simulink model "dexter_dsp_tx"  (R2020a)
settings: Solver=VariableStepAuto  StartTime=0.0  StopTime=5e4/clk  RelTol=1e-3
InitFcn:
  | dexter_dsp_init
values from neighbouring files (symbols this model uses):
  a_stimulus = [0.5 0.00 0.000]    [dexter_dsp_init.m]
  clk = 163.84e6    (= 163840000)    [dexter_dsp_init.m]
  f_stimulus = [100000 700000 768000]    [dexter_dsp_init.m]
  fs_dab = 2048e3    (= 2048000)    [dexter_dsp_init.m]
  fs_dac = clk/2    (= 81920000)    [dexter_dsp_init.m]
  interp = fir_interpolation*hb_interpolation    (= 40)    [dexter_dsp_init.m]
  tx_inc = mod(round(tx_dds_freq*2^dds_phasewidth/clk*2),2^dds_phasewidth)    [dexter_dsp_init.m]
undefined symbols (not defined in the file or in its folder): AXI4, Lite
libraries: xbsIndex_r4 x210, dspsrcs4 x1
(part 1 of 3)
settings Model: Creator=zta1  LastModifiedBy=zta1

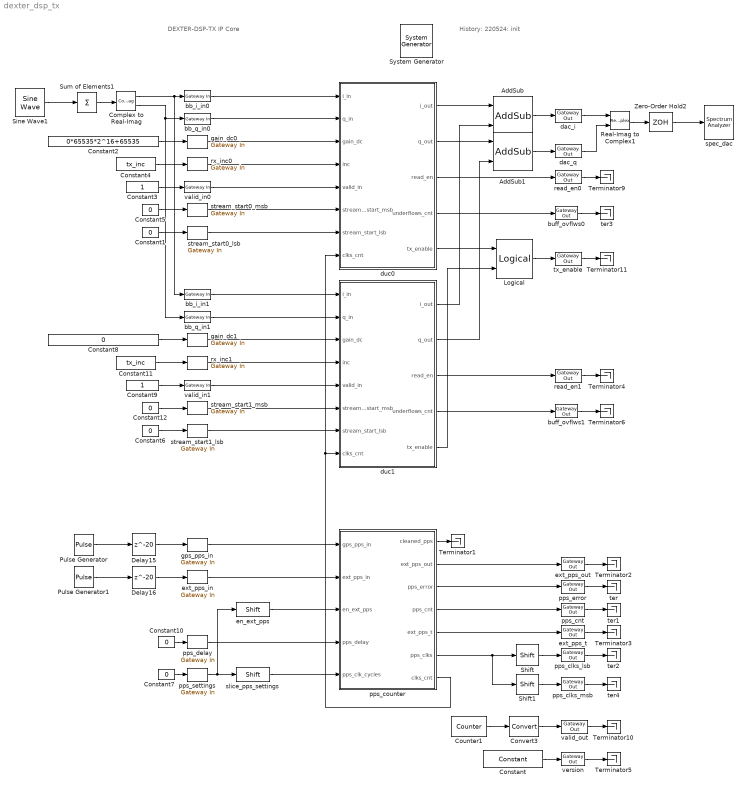
== system dexter_dsp_tx ==
  note: History:
      | 220524: init
  note: DEXTER-DSP-TX IP Core
  " System Generator" : xbsIndex_r4/ System Generator  Tag=genX  xilinxfamily=zynq  part=xc7z020  speed=-2  package=clg400  synthesis_tool=Vivado  clock_wrapper=Clock Enables  directory=../library/dexter_dsp_tx  proj_type=Vivado  Synth_file=Vivado Synthesis Defaults  Impl_file=Vivado Implementation Defaults  testbench=off  simulink_period=1/clk  sysclk_period=1e9/clk  dcm_input_clock_period=10  incr_netlist=off  trim_vbits=Everywhere in SubSystem  dbl_ovrd=According to Block Masks  core_generation=According to Block Masks  run_coregen=off  deprecated_control=off  eval_field=0  block_type=sysgen
  AddSub : xbsIndex_r4/AddSub  mode=Addition  use_carryin=off  use_carryout=off  en=off  latency=3  precision=User Defined  arith_type="Signed  (2's comp)"  n_bits=18  bin_pt=17  quantization="Round  (unbiased: +/- Inf)"  overflow=Saturate  use_behavioral_HDL=off  hw_selection=Fabric  pipelined=off  dbl_ovrd=off  block_type=addsub
  AddSub1 : xbsIndex_r4/AddSub  mode=Addition  use_carryin=off  use_carryout=off  en=off  latency=3  precision=User Defined  arith_type="Signed  (2's comp)"  n_bits=18  bin_pt=17  quantization="Round  (unbiased: +/- Inf)"  overflow=Saturate  use_behavioral_HDL=off  hw_selection=Fabric  pipelined=off  dbl_ovrd=off  block_type=addsub
  Complex to Real-Imag : ComplexToRealImag
  Constant : xbsIndex_r4/Constant  const=220524  gui_display_data_type=Fixed-point  arith_type=Unsigned  n_bits=32  bin_pt=0  preci_type=Single  exp_width=8  frac_width=24  explicit_period=on  period=1/clk  equ=P=C  opselect=C  inp2=PCIN>>17  opr=+  inp1=P  carry=CIN  dbl_ovrd=off  block_type=constant
  Constant{1,5..7,10,12} (6 alike) : Constant  Value=0  OutDataTypeStr=fixdt(0,32,0)
  Constant11 : Constant  Value=tx_inc
  Constant2 : Constant  Value=0*65535*2^16+65535  OutDataTypeStr=uint32
  Constant3 : Constant
  Constant4 : Constant  Value=tx_inc
  Constant8 : Constant  Value=0  OutDataTypeStr=uint32
  Constant9 : Constant
  Convert3 : xbsIndex_r4/Convert  gui_display_data_type=Boolean  arith_type=Boolean  n_bits=1  bin_pt=0  float_type=Single  exp_bits=8  fraction_bits=24  quantization=Truncate  overflow=Wrap  en=off  latency=0  pipeline=off  dbl_ovrd=off  block_type=convert
  Counter1 : xbsIndex_r4/Counter  cnt_type=Free Running  cnt_to=Inf  operation=Up  start_count=0  cnt_by_val=1  arith_type=Unsigned  n_bits=1  bin_pt=0  load_pin=off  rst=off  en=off  explicit_period=on  period=1/clk  use_behavioral_HDL=off  implementation=Fabric  dbl_ovrd=off  block_type=counter
  Delay15 : Delay  DelayLength=20
  Delay16 : Delay  DelayLength=20
  Logical : xbsIndex_r4/Logical  logical_function=OR  inputs=2  en=off  latency=1  precision=Full  arith_type=Unsigned  n_bits=16  bin_pt=0  align_bp=on  dbl_ovrd=off  block_type=logical
  Pulse Generator : DiscretePulseGenerator  Period=500  PulseWidth=5  SampleTime=1/clk
  Pulse Generator1 : DiscretePulseGenerator  Period=200  PulseWidth=5  SampleTime=1/clk
  Real-Imag to Complex1 : RealImagToComplex
  Shift : xbsIndex_r4/Shift  shift_dir=Right  shift_bits=0  en=off  latency=1  precision=User Defined  arith_type=Unsigned  n_bits=32  bin_pt=0  quantization=Truncate  overflow=Wrap  dbl_ovrd=off  block_type=shift
  Shift1 : xbsIndex_r4/Shift  shift_dir=Right  shift_bits=32  en=off  latency=1  precision=User Defined  arith_type=Unsigned  n_bits=32  bin_pt=0  quantization=Truncate  overflow=Wrap  dbl_ovrd=off  block_type=shift
  Sine Wave1 : dspsrcs4/Sine Wave  Amplitude=a_stimulus  Frequency=f_stimulus  Phase=0  SampleMode=Discrete  OutComplex=Complex  CompMethod=Trigonometric fcn  TableSize=Speed  SampleTime=1/fs_dab  SamplesPerFrame=1  ResetState=Restart at time zero  OutputFrames=off  dataType=double  wordLen=16  udDataType=sfix(16)  fracBitsMode=Best precision  numFracBits=15  OutDataTypeStr=double  LastOutDataTypeStr=double
  Sum of Elements1 : Sum  Inputs=+
  Terminator{1..6,9..11} (9 alike) : Terminator
  Zero-Order Hold2 : ZeroOrderHold  SampleTime=1/fs_dac
  bb_i_in0 : xbsIndex_r4/Gateway In  gui_display_data_type=Fixed-point  arith_type="Signed  (2's comp)"  n_bits=16  bin_pt=15  preci_type=Single  exp_width=8  frac_width=24  rows=1  columns=1  quantization="Round  (unbiased: +/- Inf)"  overflow=Wrap  period=1/fs_dab  UseAsADC=off  ADCChannel='1'  interface=None  automatic_assignment=on  address_offset=hex2dec('00')  intf_name=''  intf_description=''  default_value=0  timing_constraint=None  locs_specified=off  LOCs={}  io_standard={}  inherit_from_input=off  hdl_port=on  dbl_ovrd=off  block_type=gatewayin
  bb_i_in1 : xbsIndex_r4/Gateway In  gui_display_data_type=Fixed-point  arith_type="Signed  (2's comp)"  n_bits=16  bin_pt=15  preci_type=Single  exp_width=8  frac_width=24  rows=1  columns=1  quantization="Round  (unbiased: +/- Inf)"  overflow=Wrap  period=1/fs_dab  UseAsADC=off  ADCChannel='1'  interface=None  automatic_assignment=on  address_offset=hex2dec('00')  intf_name=''  intf_description=''  default_value=0  timing_constraint=None  locs_specified=off  LOCs={}  io_standard={}  inherit_from_input=off  hdl_port=on  dbl_ovrd=off  block_type=gatewayin
  bb_q_in0 : xbsIndex_r4/Gateway In  gui_display_data_type=Fixed-point  arith_type="Signed  (2's comp)"  n_bits=16  bin_pt=15  preci_type=Single  exp_width=8  frac_width=24  rows=1  columns=1  quantization="Round  (unbiased: +/- Inf)"  overflow=Wrap  period=1/fs_dab  UseAsADC=off  ADCChannel='1'  interface=None  automatic_assignment=on  address_offset=hex2dec('00')  intf_name=''  intf_description=''  default_value=0  timing_constraint=None  locs_specified=off  LOCs={}  io_standard={}  inherit_from_input=off  hdl_port=on  dbl_ovrd=off  block_type=gatewayin
  bb_q_in1 : xbsIndex_r4/Gateway In  gui_display_data_type=Fixed-point  arith_type="Signed  (2's comp)"  n_bits=16  bin_pt=15  preci_type=Single  exp_width=8  frac_width=24  rows=1  columns=1  quantization="Round  (unbiased: +/- Inf)"  overflow=Wrap  period=1/fs_dab  UseAsADC=off  ADCChannel='1'  interface=None  automatic_assignment=on  address_offset=hex2dec('00')  intf_name=''  intf_description=''  default_value=0  timing_constraint=None  locs_specified=off  LOCs={}  io_standard={}  inherit_from_input=off  hdl_port=on  dbl_ovrd=off  block_type=gatewayin
  buff_ovflws0 : xbsIndex_r4/Gateway Out  inherit_from_input=off  hdl_port=on  rows=1  columns=1  UseAsDAC=off  DACChannel='1'  interface=AXI4-Lite  automatic_assignment=off  address_offset=4*18  intf_name=''  intf_description=''  timing_constraint=None  locs_specified=off  LOCs={}  io_standard={}  block_type=gatewayout
  buff_ovflws1 : xbsIndex_r4/Gateway Out  inherit_from_input=off  hdl_port=on  rows=1  columns=1  UseAsDAC=off  DACChannel='1'  interface=AXI4-Lite  automatic_assignment=off  address_offset=4*34  intf_name=''  intf_description=''  timing_constraint=None  locs_specified=off  LOCs={}  io_standard={}  block_type=gatewayout
  dac_i : xbsIndex_r4/Gateway Out  inherit_from_input=off  hdl_port=on  rows=1  columns=1  UseAsDAC=off  DACChannel='1'  interface=None  automatic_assignment=on  address_offset=hex2dec('00')  intf_name=''  intf_description=''  timing_constraint=None  locs_specified=off  LOCs={}  io_standard={}  block_type=gatewayout
  dac_q : xbsIndex_r4/Gateway Out  inherit_from_input=off  hdl_port=on  rows=1  columns=1  UseAsDAC=off  DACChannel='1'  interface=None  automatic_assignment=on  address_offset=hex2dec('00')  intf_name=''  intf_description=''  timing_constraint=None  locs_specified=off  LOCs={}  io_standard={}  block_type=gatewayout
  duc0 : Subsystem
  duc1 : Subsystem
  en_ext_pps : xbsIndex_r4/Shift  shift_dir=Right  shift_bits=29  en=off  latency=0  precision=User Defined  arith_type=Unsigned  n_bits=1  bin_pt=0  quantization=Truncate  overflow=Wrap  dbl_ovrd=off  block_type=shift
      settings: xl_area=[0 0 0 0 0 0 0]
  ext_pps_in : xbsIndex_r4/Gateway In  gui_display_data_type=Boolean  arith_type=Boolean  n_bits=16  bin_pt=15  preci_type=Single  exp_width=8  frac_width=24  rows=1  columns=1  quantization="Round  (unbiased: +/- Inf)"  overflow=Wrap  period=1/clk  UseAsADC=off  ADCChannel='1'  interface=None  automatic_assignment=on  address_offset=hex2dec('00')  intf_name=''  intf_description=''  default_value=0  timing_constraint=None  locs_specified=off  LOCs={}  io_standard={}  inherit_from_input=off  hdl_port=on  dbl_ovrd=off  block_type=gatewayin
  ext_pps_out : xbsIndex_r4/Gateway Out  inherit_from_input=off  hdl_port=on  rows=1  columns=1  UseAsDAC=off  DACChannel='1'  interface=None  automatic_assignment=off  address_offset=10*4  intf_name=''  intf_description=''  timing_constraint=None  locs_specified=off  LOCs={}  io_standard={}  block_type=gatewayout
  ext_pps_t : xbsIndex_r4/Gateway Out  inherit_from_input=off  hdl_port=on  rows=1  columns=1  UseAsDAC=off  DACChannel='1'  interface=None  automatic_assignment=off  address_offset=10*4  intf_name=''  intf_description=''  timing_constraint=None  locs_specified=off  LOCs={}  io_standard={}  block_type=gatewayout
  gain_dc0 : xbsIndex_r4/Gateway In  gui_display_data_type=Fixed-point  arith_type=Unsigned  n_bits=32  bin_pt=0  preci_type=Single  exp_width=8  frac_width=24  rows=1  columns=1  quantization=Truncate  overflow=Wrap  period=1/fs_dab  UseAsADC=off  ADCChannel='1'  interface=AXI4-Lite  automatic_assignment=off  address_offset=4*17  intf_name=''  intf_description=''  default_value=0  timing_constraint=None  locs_specified=off  LOCs={}  io_standard={}  inherit_from_input=off  hdl_port=on  dbl_ovrd=off  block_type=gatewayin
      settings: xl_area=[0 0 0 0 32 0 0]
  gain_dc1 : xbsIndex_r4/Gateway In  gui_display_data_type=Fixed-point  arith_type=Unsigned  n_bits=32  bin_pt=0  preci_type=Single  exp_width=8  frac_width=24  rows=1  columns=1  quantization=Truncate  overflow=Wrap  period=1/fs_dab  UseAsADC=off  ADCChannel='1'  interface=AXI4-Lite  automatic_assignment=off  address_offset=4*33  intf_name=''  intf_description=''  default_value=0  timing_constraint=None  locs_specified=off  LOCs={}  io_standard={}  inherit_from_input=off  hdl_port=on  dbl_ovrd=off  block_type=gatewayin
      settings: xl_area=[0 0 0 0 32 0 0]
  gps_pps_in : xbsIndex_r4/Gateway In  gui_display_data_type=Boolean  arith_type=Boolean  n_bits=16  bin_pt=15  preci_type=Single  exp_width=8  frac_width=24  rows=1  columns=1  quantization="Round  (unbiased: +/- Inf)"  overflow=Wrap  period=1/clk  UseAsADC=off  ADCChannel='1'  interface=None  automatic_assignment=on  address_offset=hex2dec('00')  intf_name=''  intf_description=''  default_value=0  timing_constraint=None  locs_specified=off  LOCs={}  io_standard={}  inherit_from_input=off  hdl_port=on  dbl_ovrd=off  block_type=gatewayin
  pps_clks_lsb : xbsIndex_r4/Gateway Out  inherit_from_input=off  hdl_port=on  rows=1  columns=1  UseAsDAC=off  DACChannel='1'  interface=AXI4-Lite  automatic_assignment=off  address_offset=4*5  intf_name=''  intf_description=''  timing_constraint=None  locs_specified=off  LOCs={}  io_standard={}  block_type=gatewayout
  pps_clks_msb : xbsIndex_r4/Gateway Out  inherit_from_input=off  hdl_port=on  rows=1  columns=1  UseAsDAC=off  DACChannel='1'  interface=AXI4-Lite  automatic_assignment=off  address_offset=4*6  intf_name=''  intf_description=''  timing_constraint=None  locs_specified=off  LOCs={}  io_standard={}  block_type=gatewayout
  pps_cnt : xbsIndex_r4/Gateway Out  inherit_from_input=off  hdl_port=on  rows=1  columns=1  UseAsDAC=off  DACChannel='1'  interface=AXI4-Lite  automatic_assignment=off  address_offset=4*3  intf_name=''  intf_description=''  timing_constraint=None  locs_specified=off  LOCs={}  io_standard={}  block_type=gatewayout
  pps_counter : Subsystem
  pps_delay : xbsIndex_r4/Gateway In  gui_display_data_type=Fixed-point  arith_type=Unsigned  n_bits=29  bin_pt=0  preci_type=Single  exp_width=8  frac_width=24  rows=1  columns=1  quantization=Truncate  overflow=Wrap  period=1/clk  UseAsADC=off  ADCChannel='1'  interface=AXI4-Lite  automatic_assignment=off  address_offset=4*4  intf_name=''  intf_description=''  default_value=0  timing_constraint=None  locs_specified=off  LOCs={}  io_standard={}  inherit_from_input=off  hdl_port=on  dbl_ovrd=off  block_type=gatewayin
      settings: xl_area=[0 0 0 0 32 0 0]
  pps_error : xbsIndex_r4/Gateway Out  inherit_from_input=off  hdl_port=on  rows=1  columns=1  UseAsDAC=off  DACChannel='1'  interface=AXI4-Lite  automatic_assignment=off  address_offset=4*2  intf_name=''  intf_description=''  timing_constraint=None  locs_specified=off  LOCs={}  io_standard={}  block_type=gatewayout
  pps_settings : xbsIndex_r4/Gateway In  gui_display_data_type=Fixed-point  arith_type=Unsigned  n_bits=32  bin_pt=0  preci_type=Single  exp_width=8  frac_width=24  rows=1  columns=1  quantization=Truncate  overflow=Wrap  period=1/clk  UseAsADC=off  ADCChannel='1'  interface=AXI4-Lite  automatic_assignment=off  address_offset=4*1  intf_name=''  intf_description=''  default_value=0  timing_constraint=None  locs_specified=off  LOCs={}  io_standard={}  inherit_from_input=off  hdl_port=on  dbl_ovrd=off  block_type=gatewayin
      settings: xl_area=[0 0 0 0 32 0 0]
  read_en0 : xbsIndex_r4/Gateway Out  inherit_from_input=off  hdl_port=on  rows=1  columns=1  UseAsDAC=off  DACChannel='1'  interface=None  automatic_assignment=on  address_offset=hex2dec('00')  intf_name=''  intf_description=''  timing_constraint=None  locs_specified=off  LOCs={}  io_standard={}  block_type=gatewayout
  read_en1 : xbsIndex_r4/Gateway Out  inherit_from_input=off  hdl_port=on  rows=1  columns=1  UseAsDAC=off  DACChannel='1'  interface=None  automatic_assignment=on  address_offset=hex2dec('00')  intf_name=''  intf_description=''  timing_constraint=None  locs_specified=off  LOCs={}  io_standard={}  block_type=gatewayout
  rx_inc0 : xbsIndex_r4/Gateway In  gui_display_data_type=Fixed-point  arith_type=Unsigned  n_bits=dds_phasewidth  bin_pt=0  preci_type=Single  exp_width=8  frac_width=24  rows=1  columns=1  quantization=Truncate  overflow=Wrap  period=2/clk  UseAsADC=off  ADCChannel='1'  interface=AXI4-Lite  automatic_assignment=off  address_offset=4*16  intf_name=''  intf_description=''  default_value=0  timing_constraint=None  locs_specified=off  LOCs={}  io_standard={}  inherit_from_input=off  hdl_port=on  dbl_ovrd=off  block_type=gatewayin
      settings: xl_area=[0 0 0 0 32 0 0]
  rx_inc1 : xbsIndex_r4/Gateway In  gui_display_data_type=Fixed-point  arith_type=Unsigned  n_bits=dds_phasewidth  bin_pt=0  preci_type=Single  exp_width=8  frac_width=24  rows=1  columns=1  quantization=Truncate  overflow=Wrap  period=2/clk  UseAsADC=off  ADCChannel='1'  interface=AXI4-Lite  automatic_assignment=off  address_offset=4*32  intf_name=''  intf_description=''  default_value=0  timing_constraint=None  locs_specified=off  LOCs={}  io_standard={}  inherit_from_input=off  hdl_port=on  dbl_ovrd=off  block_type=gatewayin
      settings: xl_area=[0 0 0 0 32 0 0]
  slice_pps_settings : xbsIndex_r4/Shift  shift_dir=Right  shift_bits=0  en=off  latency=0  precision=User Defined  arith_type=Unsigned  n_bits=29  bin_pt=0  quantization=Truncate  overflow=Wrap  dbl_ovrd=off  block_type=shift
      settings: xl_area=[0 0 0 0 0 0 0]
  spec_dac : SpectrumAnalyzer
  stream_start0_lsb : xbsIndex_r4/Gateway In  gui_display_data_type=Fixed-point  arith_type=Unsigned  n_bits=32  bin_pt=0  preci_type=Single  exp_width=8  frac_width=24  rows=1  columns=1  quantization=Truncate  overflow=Wrap  period=1/clk  UseAsADC=off  ADCChannel='1'  interface=AXI4-Lite  automatic_assignment=off  address_offset=4*19  intf_name=''  intf_description=''  default_value=0  timing_constraint=None  locs_specified=off  LOCs={}  io_standard={}  inherit_from_input=off  hdl_port=on  dbl_ovrd=off  block_type=gatewayin
      settings: xl_area=[0 0 0 0 32 0 0]
  stream_start0_msb : xbsIndex_r4/Gateway In  gui_display_data_type=Fixed-point  arith_type=Unsigned  n_bits=32  bin_pt=0  preci_type=Single  exp_width=8  frac_width=24  rows=1  columns=1  quantization=Truncate  overflow=Wrap  period=1/clk  UseAsADC=off  ADCChannel='1'  interface=AXI4-Lite  automatic_assignment=off  address_offset=4*20  intf_name=''  intf_description=''  default_value=0  timing_constraint=None  locs_specified=off  LOCs={}  io_standard={}  inherit_from_input=off  hdl_port=on  dbl_ovrd=off  block_type=gatewayin
      settings: xl_area=[0 0 0 0 32 0 0]
  stream_start1_lsb : xbsIndex_r4/Gateway In  gui_display_data_type=Fixed-point  arith_type=Unsigned  n_bits=32  bin_pt=0  preci_type=Single  exp_width=8  frac_width=24  rows=1  columns=1  quantization=Truncate  overflow=Wrap  period=1/clk  UseAsADC=off  ADCChannel='1'  interface=AXI4-Lite  automatic_assignment=off  address_offset=4*35  intf_name=''  intf_description=''  default_value=0  timing_constraint=None  locs_specified=off  LOCs={}  io_standard={}  inherit_from_input=off  hdl_port=on  dbl_ovrd=off  block_type=gatewayin
      settings: xl_area=[0 0 0 0 32 0 0]
  stream_start1_msb : xbsIndex_r4/Gateway In  gui_display_data_type=Fixed-point  arith_type=Unsigned  n_bits=32  bin_pt=0  preci_type=Single  exp_width=8  frac_width=24  rows=1  columns=1  quantization=Truncate  overflow=Wrap  period=1/clk  UseAsADC=off  ADCChannel='1'  interface=AXI4-Lite  automatic_assignment=off  address_offset=4*36  intf_name=''  intf_description=''  default_value=0  timing_constraint=None  locs_specified=off  LOCs={}  io_standard={}  inherit_from_input=off  hdl_port=on  dbl_ovrd=off  block_type=gatewayin
      settings: xl_area=[0 0 0 0 32 0 0]
  ter{,1..4} (5 alike) : Terminator
  tx_enable : xbsIndex_r4/Gateway Out  inherit_from_input=off  hdl_port=on  rows=1  columns=1  UseAsDAC=off  DACChannel='1'  interface=None  automatic_assignment=on  address_offset=hex2dec('00')  intf_name=''  intf_description=''  timing_constraint=None  locs_specified=off  LOCs={}  io_standard={}  block_type=gatewayout
  valid_in0 : xbsIndex_r4/Gateway In  gui_display_data_type=Boolean  arith_type=Boolean  n_bits=16  bin_pt=15  preci_type=Single  exp_width=8  frac_width=24  rows=1  columns=1  quantization="Round  (unbiased: +/- Inf)"  overflow=Wrap  period=1/clk  UseAsADC=off  ADCChannel='1'  interface=None  automatic_assignment=on  address_offset=hex2dec('00')  intf_name=''  intf_description=''  default_value=0  timing_constraint=None  locs_specified=off  LOCs={}  io_standard={}  inherit_from_input=off  hdl_port=on  dbl_ovrd=off  block_type=gatewayin
  valid_in1 : xbsIndex_r4/Gateway In  gui_display_data_type=Boolean  arith_type=Boolean  n_bits=16  bin_pt=15  preci_type=Single  exp_width=8  frac_width=24  rows=1  columns=1  quantization="Round  (unbiased: +/- Inf)"  overflow=Wrap  period=1/clk  UseAsADC=off  ADCChannel='1'  interface=None  automatic_assignment=on  address_offset=hex2dec('00')  intf_name=''  intf_description=''  default_value=0  timing_constraint=None  locs_specified=off  LOCs={}  io_standard={}  inherit_from_input=off  hdl_port=on  dbl_ovrd=off  block_type=gatewayin
  valid_out : xbsIndex_r4/Gateway Out  inherit_from_input=off  hdl_port=on  rows=1  columns=1  UseAsDAC=off  DACChannel='1'  interface=None  automatic_assignment=on  address_offset=hex2dec('00')  intf_name=''  intf_description=''  timing_constraint=None  locs_specified=off  LOCs={}  io_standard={}  block_type=gatewayout
  version : xbsIndex_r4/Gateway Out  inherit_from_input=off  hdl_port=on  rows=1  columns=1  UseAsDAC=off  DACChannel='1'  interface=AXI4-Lite  automatic_assignment=off  address_offset=4*0  intf_name=''  intf_description=''  timing_constraint=None  locs_specified=off  LOCs={}  io_standard={}  block_type=gatewayout
  wires:
  version/1 -> Terminator5/1
  Constant/1 -> version/1
  Constant2/1 -> gain_dc0/1
  Sine Wave1/1 -> Sum of Elements1/1
  Sum of Elements1/1 -> Complex to Real-Imag/1
  Constant4/1 -> rx_inc0/1
  dac_i/1 -> Real-Imag to Complex1/1
  dac_q/1 -> Real-Imag to Complex1/2
  Real-Imag to Complex1/1 -> Zero-Order Hold2/1
  Zero-Order Hold2/1 -> spec_dac/1
  read_en0/1 -> Terminator9/1
  Constant3/1 -> valid_in0/1
  Convert3/1 -> valid_out/1
  Counter1/1 -> Convert3/1
  valid_out/1 -> Terminator10/1
  tx_enable/1 -> Terminator11/1
  slice_pps_settings/1 -> pps_counter/5(pps_clk_cycles)
  Constant7/1 -> pps_settings/1
  pps_delay/1 -> pps_counter/4(pps_delay)
  Pulse Generator1/1 -> Delay16/1
  gps_pps_in/1 -> pps_counter/1(gps_pps_in)
  Delay15/1 -> gps_pps_in/1
  Delay16/1 -> ext_pps_in/1
  ext_pps_in/1 -> pps_counter/2(ext_pps_in)
  Constant10/1 -> pps_delay/1
  Pulse Generator/1 -> Delay15/1
  en_ext_pps/1 -> pps_counter/3(en_ext_pps)
  pps_settings/1 -> en_ext_pps/1, slice_pps_settings/1
  pps_counter/1(cleaned_pps) -> Terminator1/1
  buff_ovflws0/1 -> ter3/1
  ext_pps_out/1 -> Terminator2/1
  pps_error/1 -> ter/1
  pps_cnt/1 -> ter1/1
  ext_pps_t/1 -> Terminator3/1
  pps_counter/6(pps_clks) -> Shift1/1, Shift/1
  pps_clks_msb/1 -> ter4/1
  Shift/1 -> pps_clks_lsb/1
  pps_clks_lsb/1 -> ter2/1
  Shift1/1 -> pps_clks_msb/1
  pps_counter/2(ext_pps_out) -> ext_pps_out/1
  pps_counter/3(pps_error) -> pps_error/1
  pps_counter/4(pps_cnt) -> pps_cnt/1
  pps_counter/5(ext_pps_t) -> ext_pps_t/1
  Constant1/1 -> stream_start0_lsb/1
  Constant5/1 -> stream_start0_msb/1
  bb_i_in0/1 -> duc0/1(i_in)
  bb_q_in0/1 -> duc0/2(q_in)
  gain_dc0/1 -> duc0/3(gain_dc)
  rx_inc0/1 -> duc0/4(inc)
  valid_in0/1 -> duc0/5(valid_in)
  stream_start0_msb/1 -> duc0/6(stream_start_msb)
  stream_start0_lsb/1 -> duc0/7(stream_start_lsb)
  duc0/1(i_out) -> AddSub/1
  duc0/3(read_en) -> read_en0/1
  duc0/4(underflows_cnt) -> buff_ovflws0/1
  duc0/5(tx_enable) -> Logical/1
  duc1/4(underflows_cnt) -> buff_ovflws1/1
  duc1/3(read_en) -> read_en1/1
  stream_start1_lsb/1 -> duc1/7(stream_start_lsb)
  stream_start1_msb/1 -> duc1/6(stream_start_msb)
  valid_in1/1 -> duc1/5(valid_in)
  rx_inc1/1 -> duc1/4(inc)
  gain_dc1/1 -> duc1/3(gain_dc)
  bb_q_in1/1 -> duc1/2(q_in)
  bb_i_in1/1 -> duc1/1(i_in)
  Constant12/1 -> stream_start1_msb/1
  Constant6/1 -> stream_start1_lsb/1
  Constant9/1 -> valid_in1/1
  Complex to Real-Imag/2 -> bb_q_in1/1, bb_q_in0/1
  Complex to Real-Imag/1 -> bb_i_in1/1, bb_i_in0/1
  Constant11/1 -> rx_inc1/1
  Constant8/1 -> gain_dc1/1
  pps_counter/7(clks_cnt) -> duc1/8(clks_cnt), duc0/8(clks_cnt)
  read_en1/1 -> Terminator4/1
  buff_ovflws1/1 -> Terminator6/1
  duc0/2(q_out) -> AddSub1/1
  AddSub1/1 -> dac_q/1
  AddSub/1 -> dac_i/1
  duc1/2(q_out) -> AddSub1/2
  duc1/1(i_out) -> AddSub/2
  duc1/5(tx_enable) -> Logical/2
  Logical/1 -> tx_enable/1

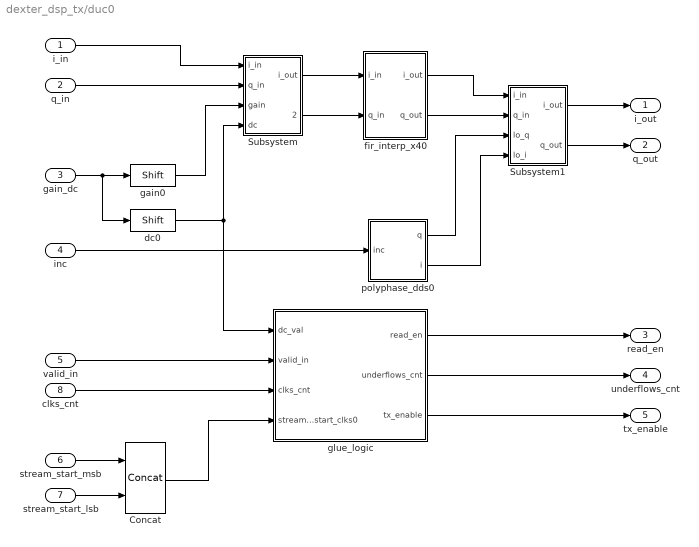
== system dexter_dsp_tx/duc0 ==
  i_in : Inport
  q_in : Inport  Port=2
  gain_dc : Inport  Port=3
  inc : Inport  Port=4
  valid_in : Inport  Port=5
  stream_start_msb : Inport  Port=6
  stream_start_lsb : Inport  Port=7
  clks_cnt : Inport  Port=8
  Concat : xbsIndex_r4/Concat  num_inputs=2  dbl_ovrd=off  block_type=concat
  Subsystem : Subsystem
  Subsystem1 : Subsystem
  dc0 : xbsIndex_r4/Shift  shift_dir=Right  shift_bits=16  en=off  latency=0  precision=User Defined  arith_type=Unsigned  n_bits=16  bin_pt=0  quantization=Truncate  overflow=Wrap  dbl_ovrd=off  block_type=shift
  fir_interp_x40 : Subsystem
  gain0 : xbsIndex_r4/Shift  shift_dir=Right  shift_bits=0  en=off  latency=0  precision=User Defined  arith_type=Unsigned  n_bits=16  bin_pt=0  quantization=Truncate  overflow=Wrap  dbl_ovrd=off  block_type=shift
  glue_logic : Subsystem
  polyphase_dds0 : Subsystem
  i_out : Outport
  q_out : Outport  Port=2
  read_en : Outport  Port=3
  underflows_cnt : Outport  Port=4
  tx_enable : Outport  Port=5
  wires:
  Subsystem1/2(q_out) -> q_out/1
  q_in/1 -> Subsystem/2(q_in)
  inc/1 -> polyphase_dds0/1(inc)
  stream_start_msb/1 -> Concat/1
  gain0/1 -> Subsystem/3(gain)
  Subsystem/1(i_out) -> fir_interp_x40/1(i_in)
  glue_logic/1(read_en) -> read_en/1
  dc0/1 -> glue_logic/1(dc_val), Subsystem/4(dc)
  fir_interp_x40/2(q_out) -> Subsystem1/2(q_in)
  Subsystem/2(q_out) -> fir_interp_x40/2(q_in)
  glue_logic/2(underflows_cnt) -> underflows_cnt/1
  i_in/1 -> Subsystem/1(i_in)
  gain_dc/1 -> dc0/1, gain0/1
  valid_in/1 -> glue_logic/2(valid_in)
  fir_interp_x40/1(i_out) -> Subsystem1/1(i_in)
  polyphase_dds0/2(i) -> Subsystem1/4(lo_i)
  polyphase_dds0/1(q) -> Subsystem1/3(lo_q)
  glue_logic/3(tx_enable) -> tx_enable/1
  Concat/1 -> glue_logic/4(stream_start_clks0)
  stream_start_lsb/1 -> Concat/2
  clks_cnt/1 -> glue_logic/3(clks_cnt)
  Subsystem1/1(i_out) -> i_out/1

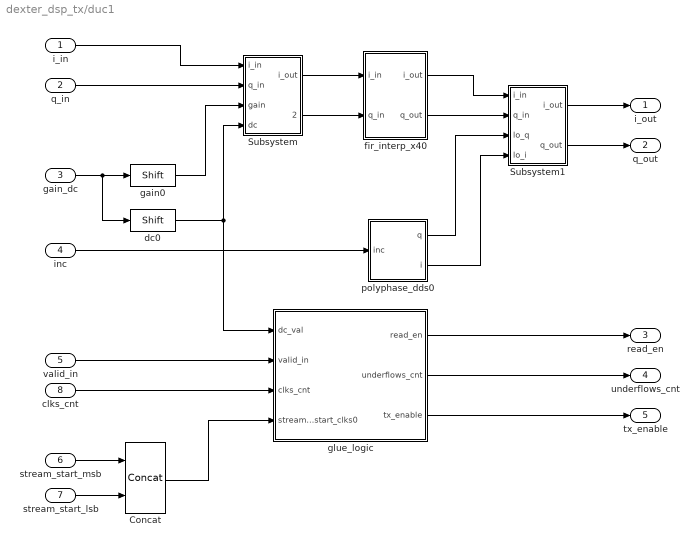
== system dexter_dsp_tx/duc1 ==
  i_in : Inport
  q_in : Inport  Port=2
  gain_dc : Inport  Port=3
  inc : Inport  Port=4
  valid_in : Inport  Port=5
  stream_start_msb : Inport  Port=6
  stream_start_lsb : Inport  Port=7
  clks_cnt : Inport  Port=8
  Concat : xbsIndex_r4/Concat  num_inputs=2  dbl_ovrd=off  block_type=concat
  Subsystem : Subsystem
  Subsystem1 : Subsystem
  dc0 : xbsIndex_r4/Shift  shift_dir=Right  shift_bits=16  en=off  latency=0  precision=User Defined  arith_type=Unsigned  n_bits=16  bin_pt=0  quantization=Truncate  overflow=Wrap  dbl_ovrd=off  block_type=shift
  fir_interp_x40 : Subsystem
  gain0 : xbsIndex_r4/Shift  shift_dir=Right  shift_bits=0  en=off  latency=0  precision=User Defined  arith_type=Unsigned  n_bits=16  bin_pt=0  quantization=Truncate  overflow=Wrap  dbl_ovrd=off  block_type=shift
  glue_logic : Subsystem
  polyphase_dds0 : Subsystem
  i_out : Outport
  q_out : Outport  Port=2
  read_en : Outport  Port=3
  underflows_cnt : Outport  Port=4
  tx_enable : Outport  Port=5
  wires:
  Subsystem1/1(i_out) -> i_out/1
  clks_cnt/1 -> glue_logic/3(clks_cnt)
  stream_start_lsb/1 -> Concat/2
  Concat/1 -> glue_logic/4(stream_start_clks0)
  glue_logic/3(tx_enable) -> tx_enable/1
  polyphase_dds0/1(q) -> Subsystem1/3(lo_q)
  polyphase_dds0/2(i) -> Subsystem1/4(lo_i)
  fir_interp_x40/1(i_out) -> Subsystem1/1(i_in)
  valid_in/1 -> glue_logic/2(valid_in)
  gain_dc/1 -> gain0/1, dc0/1
  i_in/1 -> Subsystem/1(i_in)
  glue_logic/2(underflows_cnt) -> underflows_cnt/1
  Subsystem/2(q_out) -> fir_interp_x40/2(q_in)
  fir_interp_x40/2(q_out) -> Subsystem1/2(q_in)
  dc0/1 -> Subsystem/4(dc), glue_logic/1(dc_val)
  glue_logic/1(read_en) -> read_en/1
  Subsystem/1(i_out) -> fir_interp_x40/1(i_in)
  gain0/1 -> Subsystem/3(gain)
  stream_start_msb/1 -> Concat/1
  inc/1 -> polyphase_dds0/1(inc)
  q_in/1 -> Subsystem/2(q_in)
  Subsystem1/2(q_out) -> q_out/1

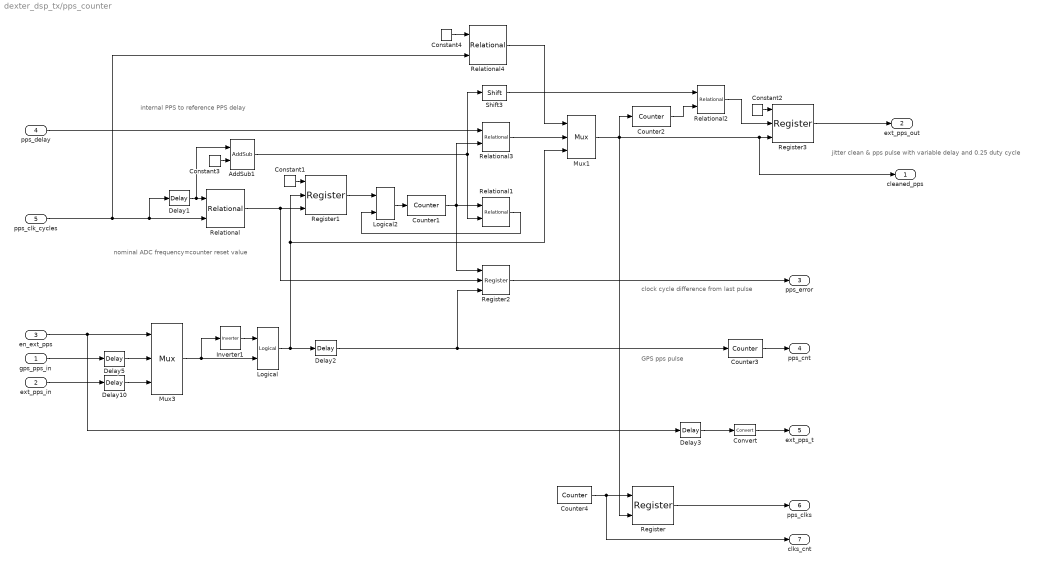
== system dexter_dsp_tx/pps_counter ==
  note: internal PPS to reference PPS delay
  note: nominal ADC frequency=counter reset value
  note: clock cycle difference from last pulse
  note: GPS pps pulse
  note: jitter clean & pps pulse with variable delay and 0.25 duty cycle
  gps_pps_in : Inport
  ext_pps_in : Inport  Port=2
  en_ext_pps : Inport  Port=3
  pps_delay : Inport  Port=4
  pps_clk_cycles : Inport  Port=5
  AddSub1 : xbsIndex_r4/AddSub  mode=Subtraction  use_carryin=off  use_carryout=off  en=off  latency=1  precision=User Defined  arith_type=Unsigned  n_bits=29  bin_pt=0  quantization=Truncate  overflow=Wrap  use_behavioral_HDL=off  hw_selection=Fabric  pipelined=off  dbl_ovrd=off  block_type=addsub
  Constant1 : xbsIndex_r4/Constant  const=1  gui_display_data_type=Boolean  arith_type=Boolean  n_bits=1  bin_pt=0  preci_type=Single  exp_width=8  frac_width=24  explicit_period=off  period=1  equ=P=C  opselect=C  inp2=PCIN>>17  opr=+  inp1=P  carry=CIN  dbl_ovrd=off  block_type=constant
  Constant2 : xbsIndex_r4/Constant  const=1  gui_display_data_type=Boolean  arith_type=Boolean  n_bits=1  bin_pt=0  preci_type=Single  exp_width=8  frac_width=24  explicit_period=off  period=1  equ=P=C  opselect=C  inp2=PCIN>>17  opr=+  inp1=P  carry=CIN  dbl_ovrd=off  block_type=constant
  Constant3 : xbsIndex_r4/Constant  const=1.0  gui_display_data_type=Fixed-point  arith_type=Unsigned  n_bits=1  bin_pt=0  preci_type=Single  exp_width=8  frac_width=24  explicit_period=off  period=1  equ=P=C  opselect=C  inp2=PCIN>>17  opr=+  inp1=P  carry=CIN  dbl_ovrd=off  block_type=constant
  Constant4 : xbsIndex_r4/Constant  const=0  gui_display_data_type=Fixed-point  arith_type=Unsigned  n_bits=1  bin_pt=0  preci_type=Single  exp_width=8  frac_width=24  explicit_period=off  period=1  equ=P=C  opselect=C  inp2=PCIN>>17  opr=+  inp1=P  carry=CIN  dbl_ovrd=off  block_type=constant
  Convert : xbsIndex_r4/Convert  gui_display_data_type=Boolean  arith_type=Boolean  n_bits=16  bin_pt=14  float_type=Single  exp_bits=8  fraction_bits=24  quantization=Truncate  overflow=Wrap  en=off  latency=0  pipeline=off  dbl_ovrd=off  block_type=convert
  Counter1 : xbsIndex_r4/Counter  cnt_type=Free Running  cnt_to=Inf  operation=Up  start_count=0  cnt_by_val=1  arith_type=Unsigned  n_bits=29  bin_pt=0  load_pin=off  rst=on  en=off  explicit_period=off  period=2  use_behavioral_HDL=off  implementation=Fabric  dbl_ovrd=off  block_type=counter
  Counter2 : xbsIndex_r4/Counter  cnt_type=Free Running  cnt_to=Inf  operation=Up  start_count=0  cnt_by_val=1  arith_type=Unsigned  n_bits=29  bin_pt=0  load_pin=off  rst=on  en=off  explicit_period=off  period=2  use_behavioral_HDL=off  implementation=Fabric  dbl_ovrd=off  block_type=counter
  Counter3 : xbsIndex_r4/Counter  cnt_type=Free Running  cnt_to=Inf  operation=Up  start_count=0  cnt_by_val=1  arith_type=Unsigned  n_bits=32  bin_pt=0  load_pin=off  rst=off  en=on  explicit_period=off  period=1/clk  use_behavioral_HDL=off  implementation=Fabric  dbl_ovrd=off  block_type=counter
  Counter4 : xbsIndex_r4/Counter  cnt_type=Free Running  cnt_to=Inf  operation=Up  start_count=0  cnt_by_val=1  arith_type=Unsigned  n_bits=64  bin_pt=0  load_pin=off  rst=off  en=off  explicit_period=on  period=1/clk  use_behavioral_HDL=off  implementation=Fabric  dbl_ovrd=off  block_type=counter
  Delay1 : xbsIndex_r4/Delay  rst=off  infoeditControl=Selection of Reset will increase slice count due to use of real FFs and instead of SRLs  en=off  latency=1  reg_retiming=off  dbl_ovrd=off  block_type=delay
  Delay10 : xbsIndex_r4/Delay  rst=off  infoeditControl=Selection of Reset will increase slice count due to use of real FFs and instead of SRLs  en=off  latency=3  reg_retiming=off  dbl_ovrd=off  block_type=delay
  Delay2 : xbsIndex_r4/Delay  rst=off  infoeditControl=Selection of Reset will increase slice count due to use of real FFs and instead of SRLs  en=off  latency=1  reg_retiming=off  dbl_ovrd=off  block_type=delay
  Delay3 : xbsIndex_r4/Delay  rst=off  infoeditControl=Selection of Reset will increase slice count due to use of real FFs and instead of SRLs  en=off  latency=1  reg_retiming=off  dbl_ovrd=off  block_type=delay
  Delay5 : xbsIndex_r4/Delay  rst=off  infoeditControl=Selection of Reset will increase slice count due to use of real FFs and instead of SRLs  en=off  latency=3  reg_retiming=off  dbl_ovrd=off  block_type=delay
  Inverter1 : xbsIndex_r4/Inverter  en=off  latency=1  dbl_ovrd=off  block_type=inv
  Logical : xbsIndex_r4/Logical  logical_function=AND  inputs=2  en=off  latency=1  precision=Full  arith_type=Unsigned  n_bits=16  bin_pt=0  align_bp=on  dbl_ovrd=off  block_type=logical
  Logical2 : xbsIndex_r4/Logical  logical_function=OR  inputs=2  en=off  latency=0  precision=Full  arith_type=Unsigned  n_bits=16  bin_pt=0  align_bp=on  dbl_ovrd=off  block_type=logical
  Mux1 : xbsIndex_r4/Mux  inputs=2  en=off  latency=0  precision=Full  arith_type=Unsigned  n_bits=16  bin_pt=14  quantization=Truncate  overflow=Wrap  dbl_ovrd=off  block_type=mux
  Mux3 : xbsIndex_r4/Mux  inputs=2  en=off  latency=1  precision=Full  arith_type=Unsigned  n_bits=16  bin_pt=14  quantization=Truncate  overflow=Wrap  dbl_ovrd=off  block_type=mux
  Register : xbsIndex_r4/Register  init=0  rst=off  en=on  dbl_ovrd=off  block_type=register
  Register1 : xbsIndex_r4/Register  init=0  rst=on  en=on  dbl_ovrd=off  block_type=register
  Register2 : xbsIndex_r4/Register  init=0  rst=on  en=on  dbl_ovrd=off  block_type=register
  Register3 : xbsIndex_r4/Register  init=0  rst=on  en=on  dbl_ovrd=off  block_type=register
  Relational : xbsIndex_r4/Relational  mode=a!=b  op_type=Bool  en=off  latency=1  dbl_ovrd=off  block_type=relational
  Relational1 : xbsIndex_r4/Relational  mode=a>=b  op_type=Bool  en=off  latency=0  dbl_ovrd=off  block_type=relational
  Relational2 : xbsIndex_r4/Relational  mode=a=b  op_type=Bool  en=off  latency=1  dbl_ovrd=off  block_type=relational
  Relational3 : xbsIndex_r4/Relational  mode=a=b  op_type=Bool  en=off  latency=1  dbl_ovrd=off  block_type=relational
  Relational4 : xbsIndex_r4/Relational  mode=a=b  op_type=Ufix  en=off  latency=1  dbl_ovrd=off  block_type=relational
  Shift3 : xbsIndex_r4/Shift  shift_dir=Right  shift_bits=3  en=off  latency=0  precision=User Defined  arith_type=Unsigned  n_bits=29  bin_pt=0  quantization=Truncate  overflow=Wrap  dbl_ovrd=off  block_type=shift
  cleaned_pps : Outport
  ext_pps_out : Outport  Port=2
  pps_error : Outport  Port=3
  pps_cnt : Outport  Port=4
  ext_pps_t : Outport  Port=5
  pps_clks : Outport  Port=6
  clks_cnt : Outport  Port=7
  wires:
  Mux3/1 -> Inverter1/1, Logical/2
  gps_pps_in/1 -> Delay5/1
  Inverter1/1 -> Logical/1
  Logical/1 -> Delay2/1, Mux1/3, Register1/2
  ext_pps_in/1 -> Delay10/1
  Delay5/1 -> Mux3/2
  en_ext_pps/1 -> Delay3/1, Mux3/1
  Delay10/1 -> Mux3/3
  pps_clk_cycles/1 -> Relational4/2, Delay1/1, Relational/2
  Delay1/1 -> AddSub1/1, Relational/1
  Constant1/1 -> Register1/1
  Relational/1 -> Register1/3, Register2/2
  Logical2/1 -> Counter1/1
  Register1/1 -> Logical2/1
  Counter1/1 -> Relational1/1, Register2/1, Relational3/2
  Constant3/1 -> AddSub1/2
  AddSub1/1 -> Shift3/1, Relational1/2
  Relational1/1 -> Logical2/2
  Delay2/1 -> Counter3/1, Register2/3
  Constant2/1 -> Register3/1
  Shift3/1 -> Relational2/1
  Mux1/1 -> Register/2, cleaned_pps/1, Register3/3, Counter2/1
  pps_delay/1 -> Relational3/1
  Counter2/1 -> Relational2/2
  Relational2/1 -> Register3/2
  Counter3/1 -> pps_cnt/1
  Register2/1 -> pps_error/1
  Register3/1 -> ext_pps_out/1
  Convert/1 -> ext_pps_t/1
  Delay3/1 -> Convert/1
  Relational3/1 -> Mux1/2
  Constant4/1 -> Relational4/1
  Relational4/1 -> Mux1/1
  Counter4/1 -> clks_cnt/1, Register/1
  Register/1 -> pps_clks/1

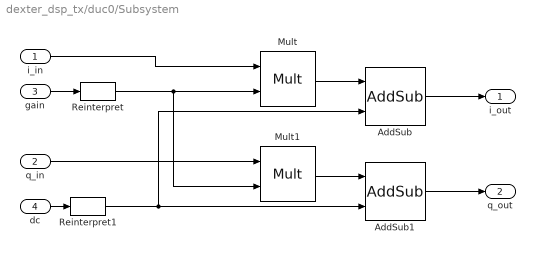
== system dexter_dsp_tx/duc0/Subsystem ==
  i_in : Inport
  q_in : Inport  Port=2
  gain : Inport  Port=3
  dc : Inport  Port=4
  AddSub : xbsIndex_r4/AddSub  mode=Addition  use_carryin=off  use_carryout=off  en=off  latency=1  precision=User Defined  arith_type="Signed  (2's comp)"  n_bits=16  bin_pt=15  quantization=Truncate  overflow=Wrap  use_behavioral_HDL=off  hw_selection=Fabric  pipelined=off  dbl_ovrd=off  block_type=addsub
  AddSub1 : xbsIndex_r4/AddSub  mode=Addition  use_carryin=off  use_carryout=off  en=off  latency=1  precision=User Defined  arith_type="Signed  (2's comp)"  n_bits=16  bin_pt=15  quantization=Truncate  overflow=Wrap  use_behavioral_HDL=off  hw_selection=Fabric  pipelined=off  dbl_ovrd=off  block_type=addsub
  Mult : xbsIndex_r4/Mult  precision=User Defined  arith_type="Signed  (2's comp)"  n_bits=16  bin_pt=15  quantization="Round  (unbiased: +/- Inf)"  overflow=Wrap  en=off  latency=4  use_behavioral_HDL=off  opt=Speed  use_embedded=on  optimum_pipeline=off  pipeline=on  dbl_ovrd=off  use_rpm=on  placement_style=Triangular  block_type=mult
  Mult1 : xbsIndex_r4/Mult  precision=User Defined  arith_type="Signed  (2's comp)"  n_bits=16  bin_pt=15  quantization="Round  (unbiased: +/- Inf)"  overflow=Wrap  en=off  latency=4  use_behavioral_HDL=off  opt=Speed  use_embedded=on  optimum_pipeline=off  pipeline=on  dbl_ovrd=off  use_rpm=on  placement_style=Triangular  block_type=mult
  Reinterpret : xbsIndex_r4/Reinterpret  force_arith_type=on  arith_type=Unsigned  force_bin_pt=on  bin_pt=16  block_type=reinterpret
  Reinterpret1 : xbsIndex_r4/Reinterpret  force_arith_type=on  arith_type=Unsigned  force_bin_pt=on  bin_pt=16  block_type=reinterpret
  i_out : Outport
  q_out : Outport  Port=2
  wires:
  i_in/1 -> Mult/1
  Reinterpret1/1 -> AddSub/2, AddSub1/2
  gain/1 -> Reinterpret/1
  Mult1/1 -> AddSub1/1
  q_in/1 -> Mult1/1
  AddSub/1 -> i_out/1
  Mult/1 -> AddSub/1
  AddSub1/1 -> q_out/1
  dc/1 -> Reinterpret1/1
  Reinterpret/1 -> Mult1/2, Mult/2

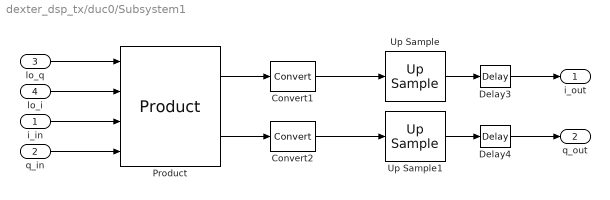
== system dexter_dsp_tx/duc0/Subsystem1 ==
  i_in : Inport
  q_in : Inport  Port=2
  lo_q : Inport  Port=3
  lo_i : Inport  Port=4
  Convert1 : xbsIndex_r4/Convert  gui_display_data_type=Fixed-point  arith_type="Signed  (2's comp)"  n_bits=18  bin_pt=17  float_type=Single  exp_bits=8  fraction_bits=24  quantization="Round  (unbiased: +/- Inf)"  overflow=Saturate  en=off  latency=1  pipeline=off  dbl_ovrd=off  block_type=convert
  Convert2 : xbsIndex_r4/Convert  gui_display_data_type=Fixed-point  arith_type="Signed  (2's comp)"  n_bits=18  bin_pt=17  float_type=Single  exp_bits=8  fraction_bits=24  quantization="Round  (unbiased: +/- Inf)"  overflow=Saturate  en=off  latency=1  pipeline=off  dbl_ovrd=off  block_type=convert
  Delay3 : xbsIndex_r4/Delay  rst=off  infoeditControl=Selection of Reset will increase slice count due to use of real FFs and instead of SRLs  en=off  latency=2  reg_retiming=off  dbl_ovrd=off  block_type=delay
  Delay4 : xbsIndex_r4/Delay  rst=off  infoeditControl=Selection of Reset will increase slice count due to use of real FFs and instead of SRLs  en=off  latency=2  reg_retiming=off  dbl_ovrd=off  block_type=delay
  Product : xbsIndex_r4/Product  complex_multiplier=on  optimizegoal=Performance  simulation_type=fast_sim  simulation_model=sysgen:product_macro  block_type=product_macro
  Up Sample : xbsIndex_r4/Up Sample  sample_ratio=2  copy_samples=on  en=off  latency=1  dbl_ovrd=off  block_type=usamp
  Up Sample1 : xbsIndex_r4/Up Sample  sample_ratio=2  copy_samples=on  en=off  latency=1  dbl_ovrd=off  block_type=usamp
  i_out : Outport
  q_out : Outport  Port=2
  wires:
  q_in/1 -> Product/4
  i_in/1 -> Product/3
  Product/2 -> Convert2/1
  Convert1/1 -> Up Sample/1
  lo_i/1 -> Product/2
  Up Sample/1 -> Delay3/1
  Convert2/1 -> Up Sample1/1
  Delay4/1 -> q_out/1
  lo_q/1 -> Product/1
  Up Sample1/1 -> Delay4/1
  Delay3/1 -> i_out/1
  Product/1 -> Convert1/1
